simulink model "Dc_motor_control"  (R2015a)
settings: Solver=ode45  StartTime=0.0  StopTime=10.0  RelTol=1e-3
libraries: cstblocks x1
settings Model: Creator=Eduardo A Herrera  LastModifiedBy=Eduardo A Herrera

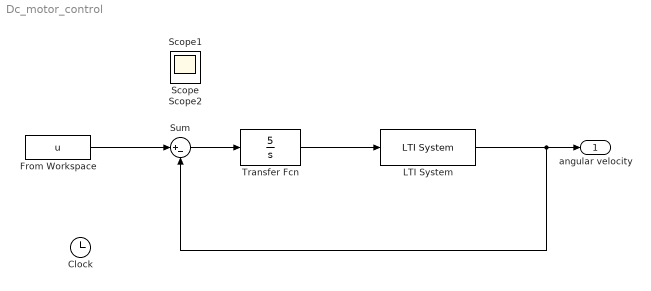
== system Dc_motor_control ==
  Clock : Clock
  From Workspace : FromWorkspace  VariableName=u  SampleTime=0
  LTI System : cstblocks/LTI System  sys=dcm  IC=[]
  Sum : Sum  Inputs=|+-  OutMin=[1]  OutMax=1
  Transfer Fcn : TransferFcn  Numerator=[5]  Denominator=[1 0]
  angular velocity : Outport
  Scope : Scope
  Scope1 : Scope
  Scope2 : Scope
      settings: SaveName=ScopeData2
  wires:
  From Workspace/1 -> Sum/1
  Transfer Fcn/1 -> LTI System/1
  Sum/1 -> Transfer Fcn/1
  LTI System/1 -> Sum/2, angular velocity/1
